simulink model "TBRe19_ECU_SequentialTests"  (R2017b)
settings: Solver=FixedStepDiscrete  StartTime=0.0  StopTime=inf  FixedStep=0.0001  RelTol=1e-3
PostLoadFcn:
  | model_init();
libraries: simulink x28
(part 22 of 22)

== matlab function TBRe19_ECU_SequentialTests/PedalBox/Pre_Processing_Layer/Pedal_Box/Sensor Plausibility/Sensor_Diag ==
  data: TV_1 input; Pedal_Sensor_Fail output; TV_2 input; BV_POT input; TV1_Out output; TV2_Out output; BV_1 input; BVPot_Out output; BV_2 input; BV1_Out output; BV2_Out output
function [Pedal_Sensor_Fail,TV1_Out,TV2_Out,BVPot_Out, BV1_Out, BV2_Out ] = Sensor_Diagnostics(TV_1,TV_2,BV_POT , BV_1, BV_2)
%Checks whether the throttle sensors are in their calibrated range

%Initialisation of throttle outputs, default low 
TV1_Out=uint16(0);
TV2_Out=uint16(0);
BVPot_Out=uint16(0);
BV1_Out=uint16(0);
BV2_Out=uint16(0);

Pedal_Sensor_Fail = uint8(0);

if (TV_1>10000 || TV_1<000) %if V1 out of normal range
    Pedal_Sensor_Fail = Pedal_Sensor_Fail + uint8(1);
   
end

if (TV_2>10000 || TV_2<0000) %if V2 out of normal range
    Pedal_Sensor_Fail = Pedal_Sensor_Fail + uint8(2);
end   

if (BV_POT>17000 || BV_POT<0) %if brake out of normal range
    Pedal_Sensor_Fail = Pedal_Sensor_Fail + uint8(4);
  
end

if (BV_POT>17000 || BV_POT<0) %if brake out of normal range
    Pedal_Sensor_Fail = Pedal_Sensor_Fail + uint8(8);
  
end

if (BV_POT>17000 || BV_POT<0) %if brake out of normal range
    Pedal_Sensor_Fail = Pedal_Sensor_Fail + uint8(16);
  
end

if(Pedal_Sensor_Fail == 0) %if no error pass voltages to pedal checks
    TV1_Out=uint16(TV_1);
    TV2_Out=uint16(TV_2);
    BVPot_Out=uint16(BV_POT);
    BV1_Out = uint16(BV_1);
    BV2_Out = uint16(BV_2);
end

== stateflow chart TBRe19_ECU_SequentialTests/FullPrePLandCoolant/Post_Processing_Layer/Dash_LEDs/Flashy ==
  state Init
    entry:
    Light = true;
  state Normal
    entry:
    Light = false;
  (default) -> Init
  Init -> Normal : after(0.5,sec)
  Normal -> Init : after(0.5,sec)
  data: Light output boolean =true

== stateflow chart TBRe19_ECU_SequentialTests/FullPrePLandCoolant/Post_Processing_Layer/Dash_LEDs/InitLight ==
  state Init
    entry:
    Light = true;
  state Normal
    entry:
    Light = false;
  (default) -> Init
  Init -> Normal : after(2.5,sec)
  data: Light output boolean =true

== stateflow chart TBRe19_ECU_SequentialTests/FullPrePLandCoolant/Post_Processing_Layer/Dash_LEDs/Wake_Up ==
  state Init
    entry:
    RTD = true;
    X = false;
    Y = false;
    Z = false;
  state One
    entry:
    RTD = false;
    X = true;
    Y = false;
    Z = false;
  state Two
    entry:
    RTD = false;
    X = false;
    Y = true;
    Z = false;
  state Three
    entry:
    RTD = false;
    X = false;
    Y = false;
    Z = true;
  state Normal
    entry:
    RTD = false;
    X = false;
    Y = false;
    Z = false;
  (default) -> Init
  Init -> One : after(0.5,sec)
  One -> Two : after(0.5,sec)
  Two -> Three : after(0.5, sec)
  Three -> Normal : after(0.5, sec)
  data: RTD output boolean =true; X output boolean =true; Y output boolean =true; Z output boolean =true

== matlab function TBRe19_ECU_SequentialTests/FullPrePLandCoolant/Pre_Processing_Layer/Pedal_Box/Sensor Plausibility/Sensor_Diag ==
  data: TV_1 input; Pedal_Sensor_Fail output; TV_2 input; BV_POT input; TV1_Out output; TV2_Out output; BV_1 input; BVPot_Out output; BV_2 input; BV1_Out output; BV2_Out output
function [Pedal_Sensor_Fail,TV1_Out,TV2_Out,BVPot_Out, BV1_Out, BV2_Out ] = Sensor_Diagnostics(TV_1,TV_2,BV_POT , BV_1, BV_2)
%Checks whether the throttle sensors are in their calibrated range

%Initialisation of throttle outputs, default low 
TV1_Out=uint16(0);
TV2_Out=uint16(0);
BVPot_Out=uint16(0);
BV1_Out=uint16(0);
BV2_Out=uint16(0);

Pedal_Sensor_Fail = uint8(0);

if (TV_1>10000 || TV_1<000) %if V1 out of normal range
    Pedal_Sensor_Fail = Pedal_Sensor_Fail + uint8(1);
   
end

if (TV_2>10000 || TV_2<0000) %if V2 out of normal range
    Pedal_Sensor_Fail = Pedal_Sensor_Fail + uint8(2);
end   

if (BV_POT>17000 || BV_POT<0) %if brake out of normal range
    Pedal_Sensor_Fail = Pedal_Sensor_Fail + uint8(4);
  
end

if (BV_POT>17000 || BV_POT<0) %if brake out of normal range
    Pedal_Sensor_Fail = Pedal_Sensor_Fail + uint8(8);
  
end

if (BV_POT>17000 || BV_POT<0) %if brake out of normal range
    Pedal_Sensor_Fail = Pedal_Sensor_Fail + uint8(16);
  
end

if(Pedal_Sensor_Fail == 0) %if no error pass voltages to pedal checks
    TV1_Out=uint16(TV_1);
    TV2_Out=uint16(TV_2);
    BVPot_Out=uint16(BV_POT);
    BV1_Out = uint16(BV_1);
    BV2_Out = uint16(BV_2);
end

== stateflow chart TBRe19_ECU_SequentialTests/RTDandStateMachine/Post_Processing_Layer/Dash_LEDs/Flashy ==
  state Init
    entry:
    Light = true;
  state Normal
    entry:
    Light = false;
  (default) -> Init
  Init -> Normal : after(0.5,sec)
  Normal -> Init : after(0.5,sec)
  data: Light output boolean =true

== stateflow chart TBRe19_ECU_SequentialTests/RTDandStateMachine/Post_Processing_Layer/Dash_LEDs/InitLight ==
  state Init
    entry:
    Light = true;
  state Normal
    entry:
    Light = false;
  (default) -> Init
  Init -> Normal : after(2.5,sec)
  data: Light output boolean =true

== stateflow chart TBRe19_ECU_SequentialTests/RTDandStateMachine/Post_Processing_Layer/Dash_LEDs/Wake_Up ==
  state Init
    entry:
    RTD = true;
    X = false;
    Y = false;
    Z = false;
  state One
    entry:
    RTD = false;
    X = true;
    Y = false;
    Z = false;
  state Two
    entry:
    RTD = false;
    X = false;
    Y = true;
    Z = false;
  state Three
    entry:
    RTD = false;
    X = false;
    Y = false;
    Z = true;
  state Normal
    entry:
    RTD = false;
    X = false;
    Y = false;
    Z = false;
  (default) -> Init
  Init -> One : after(0.5,sec)
  One -> Two : after(0.5,sec)
  Two -> Three : after(0.5, sec)
  Three -> Normal : after(0.5, sec)
  data: RTD output boolean =true; X output boolean =true; Y output boolean =true; Z output boolean =true

== matlab function TBRe19_ECU_SequentialTests/RTDandStateMachine/Pre_Processing_Layer/Pedal_Box/Sensor Plausibility/Sensor_Diag ==
  data: TV_1 input; Pedal_Sensor_Fail output; TV_2 input; BV_POT input; TV1_Out output; TV2_Out output; BV_1 input; BVPot_Out output; BV_2 input; BV1_Out output; BV2_Out output
function [Pedal_Sensor_Fail,TV1_Out,TV2_Out,BVPot_Out, BV1_Out, BV2_Out ] = Sensor_Diagnostics(TV_1,TV_2,BV_POT , BV_1, BV_2)
%Checks whether the throttle sensors are in their calibrated range

%Initialisation of throttle outputs, default low 
TV1_Out=uint16(0);
TV2_Out=uint16(0);
BVPot_Out=uint16(0);
BV1_Out=uint16(0);
BV2_Out=uint16(0);

Pedal_Sensor_Fail = uint8(0);

if (TV_1>10000 || TV_1<000) %if V1 out of normal range
    Pedal_Sensor_Fail = Pedal_Sensor_Fail + uint8(1);
   
end

if (TV_2>10000 || TV_2<0000) %if V2 out of normal range
    Pedal_Sensor_Fail = Pedal_Sensor_Fail + uint8(2);
end   

if (BV_POT>17000 || BV_POT<0) %if brake out of normal range
    Pedal_Sensor_Fail = Pedal_Sensor_Fail + uint8(4);
  
end

if (BV_POT>17000 || BV_POT<0) %if brake out of normal range
    Pedal_Sensor_Fail = Pedal_Sensor_Fail + uint8(8);
  
end

if (BV_POT>17000 || BV_POT<0) %if brake out of normal range
    Pedal_Sensor_Fail = Pedal_Sensor_Fail + uint8(16);
  
end

if(Pedal_Sensor_Fail == 0) %if no error pass voltages to pedal checks
    TV1_Out=uint16(TV_1);
    TV2_Out=uint16(TV_2);
    BVPot_Out=uint16(BV_POT);
    BV1_Out = uint16(BV_1);
    BV2_Out = uint16(BV_2);
end

== stateflow chart TBRe19_ECU_SequentialTests/RTDandStateMachine/Vehicle_Functionality_Layer/Vehicle_Operation_Mode/Operaton_Mode ==
  note: Start here
  state Standby_State
    entry:
    Control_Word = uint8(0); %Off
    MCU_NMT_Mode = uint8(2); %Pre-Operational Mode
    State = 1;
  state Error_State
    entry:
    Control_Word = uint8(6); %Error
    MCU_NMT_Mode = uint8(0); %Stopped Mode
    State = 0;
  note: (ECU errors)
  note: btnRTD is for rules
      | TSS is for our safety
  state RTD_State
    entry:
    Control_Word = uint8(5); %ReadyToDrive
    MCU_NMT_Mode = uint8(3); %Operational Mode
    State = 3;
  state Buzzer_State
    entry:
    Control_Word = uint8(3); %Energise
    MCU_NMT_Mode = uint8(2); %Pre-Operational Mode
    State = 2;
  (default) -> Error_State
  Error_State -> Standby_State : [~Error]
  Standby_State -> Error_State [order 1] : [Error]
  RTD_State -> Standby_State [order 2] : [btnRTD || ~TSS]
  RTD_State -> Error_State [order 1] : [Error]
  Buzzer_State -> Error_State [order 1] : [Error]
  Standby_State -> Buzzer_State [order 2] : [btnRTD && Brake && ~Throttle && TSS]
  Buzzer_State -> RTD_State [order 2] : after(1.5,sec)
  data: MCU_NMT_Mode output uint8; Control_Word output uint8; State output uint8; Throttle input boolean; Brake input boolean; btnRTD input boolean; btnRTD_Hold input boolean; Error input boolean; TSS input boolean

== stateflow chart TBRe19_ECU_SequentialTests/DriveFunction/Post_Processing_Layer/Dash_LEDs/Flashy ==
  state Init
    entry:
    Light = true;
  state Normal
    entry:
    Light = false;
  (default) -> Init
  Init -> Normal : after(0.5,sec)
  Normal -> Init : after(0.5,sec)
  data: Light output boolean =true

== stateflow chart TBRe19_ECU_SequentialTests/DriveFunction/Post_Processing_Layer/Dash_LEDs/InitLight ==
  state Init
    entry:
    Light = true;
  state Normal
    entry:
    Light = false;
  (default) -> Init
  Init -> Normal : after(2.5,sec)
  data: Light output boolean =true

== stateflow chart TBRe19_ECU_SequentialTests/DriveFunction/Post_Processing_Layer/Dash_LEDs/Wake_Up ==
  state Init
    entry:
    RTD = true;
    X = false;
    Y = false;
    Z = false;
  state One
    entry:
    RTD = false;
    X = true;
    Y = false;
    Z = false;
  state Two
    entry:
    RTD = false;
    X = false;
    Y = true;
    Z = false;
  state Three
    entry:
    RTD = false;
    X = false;
    Y = false;
    Z = true;
  state Normal
    entry:
    RTD = false;
    X = false;
    Y = false;
    Z = false;
  (default) -> Init
  Init -> One : after(0.5,sec)
  One -> Two : after(0.5,sec)
  Two -> Three : after(0.5, sec)
  Three -> Normal : after(0.5, sec)
  data: RTD output boolean =true; X output boolean =true; Y output boolean =true; Z output boolean =true

== matlab function TBRe19_ECU_SequentialTests/DriveFunction/Pre_Processing_Layer/Pedal_Box/Sensor Plausibility/Sensor_Diag ==
  data: TV_1 input; Pedal_Sensor_Fail output; TV_2 input; BV_POT input; TV1_Out output; TV2_Out output; BV_1 input; BVPot_Out output; BV_2 input; BV1_Out output; BV2_Out output
function [Pedal_Sensor_Fail,TV1_Out,TV2_Out,BVPot_Out, BV1_Out, BV2_Out ] = Sensor_Diagnostics(TV_1,TV_2,BV_POT , BV_1, BV_2)
%Checks whether the throttle sensors are in their calibrated range

%Initialisation of throttle outputs, default low 
TV1_Out=uint16(0);
TV2_Out=uint16(0);
BVPot_Out=uint16(0);
BV1_Out=uint16(0);
BV2_Out=uint16(0);

Pedal_Sensor_Fail = uint8(0);

if (TV_1>10000 || TV_1<000) %if V1 out of normal range
    Pedal_Sensor_Fail = Pedal_Sensor_Fail + uint8(1);
   
end

if (TV_2>10000 || TV_2<0000) %if V2 out of normal range
    Pedal_Sensor_Fail = Pedal_Sensor_Fail + uint8(2);
end   

if (BV_POT>17000 || BV_POT<0) %if brake out of normal range
    Pedal_Sensor_Fail = Pedal_Sensor_Fail + uint8(4);
  
end

if (BV_POT>17000 || BV_POT<0) %if brake out of normal range
    Pedal_Sensor_Fail = Pedal_Sensor_Fail + uint8(8);
  
end

if (BV_POT>17000 || BV_POT<0) %if brake out of normal range
    Pedal_Sensor_Fail = Pedal_Sensor_Fail + uint8(16);
  
end

if(Pedal_Sensor_Fail == 0) %if no error pass voltages to pedal checks
    TV1_Out=uint16(TV_1);
    TV2_Out=uint16(TV_2);
    BVPot_Out=uint16(BV_POT);
    BV1_Out = uint16(BV_1);
    BV2_Out = uint16(BV_2);
end

== matlab function TBRe19_ECU_SequentialTests/DriveFunction/Vehicle_Functionality_Layer/Drive_Function/Regen_Braking/Torque_Mode ==
  data: Throttle input; Torque output; Brake input; Coast input; Speed input; RegenOk input; RegenBool output
function [Torque, RegenBool]= fcn(Throttle, Brake, Coast,Speed,RegenOk )
%Set Torque depending on drive, coas of braking
Coast = int16(Coast);


if(Throttle > 0)
    %Driving Demand
    Torque = int16(Throttle);
elseif(Throttle == 0 && Brake  == 0)
    %Vehicle is coasting
    Torque = int16(Coast);
elseif(Brake > 0)
    %Vehicle is braking
    Torque = int16(Brake);
else
    %Safety
    Torque = int16(0);
end

if (RegenOk == false && Torque < 0)
    Torque  = int16(0);
elseif (Speed < 1.5 && Torque < 0) %5km/h rule is 1.4 m/s
    Torque  = int16(0);
    %Don't regen when vehicle is stationary 
else
    Torque = int16(Torque);
    %nothing
end


if(Torque < 0)
    RegenBool = true;
else
    RegenBool = false;
end

== stateflow chart TBRe19_ECU_SequentialTests/DriveFunction/Vehicle_Functionality_Layer/Vehicle_Operation_Mode/Operaton_Mode ==
  note: Start here
  state Standby_State
    entry:
    Control_Word = uint8(0); %Off
    MCU_NMT_Mode = uint8(2); %Pre-Operational Mode
    State = 1;
  state Error_State
    entry:
    Control_Word = uint8(6); %Error
    MCU_NMT_Mode = uint8(0); %Stopped Mode
    State = 0;
  note: (ECU errors)
  note: btnRTD is for rules
      | TSS is for our safety
  state RTD_State
    entry:
    Control_Word = uint8(5); %ReadyToDrive
    MCU_NMT_Mode = uint8(3); %Operational Mode
    State = 3;
  state Buzzer_State
    entry:
    Control_Word = uint8(3); %Energise
    MCU_NMT_Mode = uint8(2); %Pre-Operational Mode
    State = 2;
  (default) -> Error_State
  Error_State -> Standby_State : [~Error]
  Standby_State -> Error_State [order 1] : [Error]
  RTD_State -> Standby_State [order 2] : [btnRTD || ~TSS]
  RTD_State -> Error_State [order 1] : [Error]
  Buzzer_State -> Error_State [order 1] : [Error]
  Standby_State -> Buzzer_State [order 2] : [btnRTD && Brake && ~Throttle && TSS]
  Buzzer_State -> RTD_State [order 2] : after(1.5,sec)
  data: MCU_NMT_Mode output uint8; Control_Word output uint8; State output uint8; Throttle input boolean; Brake input boolean; btnRTD input boolean; btnRTD_Hold input boolean; Error input boolean; TSS input boolean
